simulink library "WECSim_Lib_PTOs"  (R2020b)
settings: Solver=VariableStepAuto  StartTime=0.0  StopTime=10.0  RelTol=1e-3
undefined symbols (not defined in the file or in its folder): constraint, pto, simu, X, Y, Z
libraries: nesl_utility x71, sm_lib x46, WECSim_Lib_Body_Elements x1
(part 3 of 3)

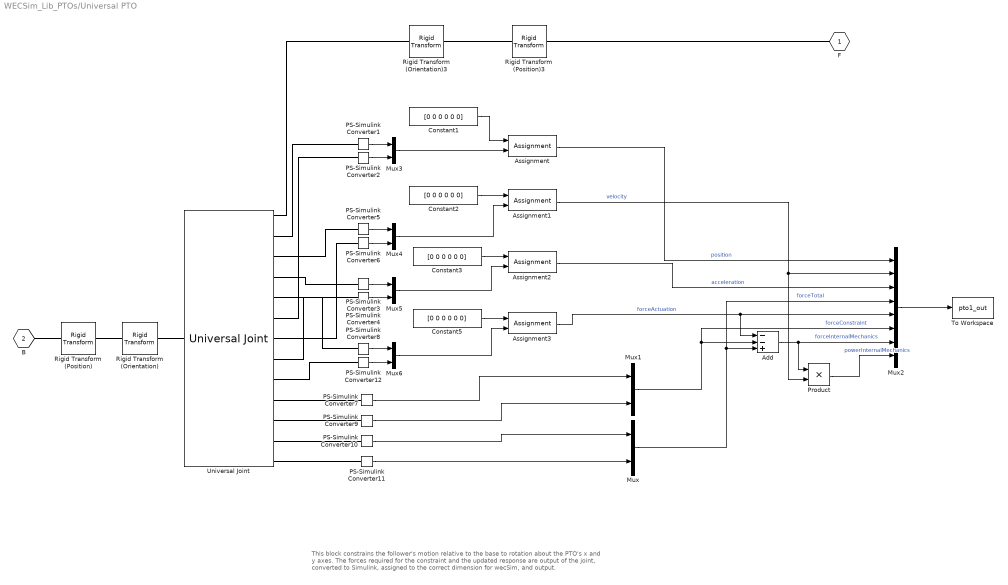
== system WECSim_Lib_PTOs/Universal PTO ==
  note: This block constrains the follower's motion relative to the base to rotation about the PTO's x and y axes. The forces required for the constraint and the updated response are output of the joint, converted to Simulink, assigned to the correct dimension for wecSim, and output.
  Add : Sum  Inputs=--+
  Assignment : Assignment  IndexOptions=Index vector (dialog)  Indices=[4 5]  OutputSizes=1
  Assignment1 : Assignment  IndexOptions=Index vector (dialog)  Indices=[4 5]  OutputSizes=1
  Assignment2 : Assignment  IndexOptions=Index vector (dialog)  Indices=[4,5]  OutputSizes=1
  Assignment3 : Assignment  IndexOptions=Index vector (dialog)  Indices=[4,5]  OutputSizes=1
  Constant{1..3,5} (4 alike) : Constant  Value=[0 0 0 0 0 0]
  Mux{,1,3..6} (6 alike) : Mux  Inputs=2
  Mux2 : Mux  Inputs=8
  PS-Simulink Converter{1..12} (12 alike) : nesl_utility/PS-Simulink Converter  PhysicalDomain=network_engine_domain  SubClassName=ps_output  LeftPortType=input  RightPortType=output  PseudoPeriodic=off  Frequencies=[]  VectorFormat=1-D array  Unit=inherit  AffineConversion=off
  Product : Product
  Rigid Transform (Orientation) : sm_lib/Frames and Transforms/Rigid Transform  RotationMethod=RotationMatrix  FollAlignAxisA=+X  BaseAlignAxisA=+Y  FollAlignAxisB=+Y  BaseAlignAxisB=+Z  RotationStandardAxis=+Z  RotationAngle=0.0  RotationAngleUnits=deg  RotationArbitraryAxis=[0 0 1]  RotationSequenceAxes=FollowerAxes  RotationSequence=XYX  RotationSequenceAngles=[0 0 0]  RotationSequenceAnglesUnits=deg  RotationMatrix=pto.orientation.rotationMatrix  Quaternion=[1 0 0 0]  TranslationMethod=None  TranslationCartesianOffset=constraint.initial.displacement+constraint.location  TranslationCartesianOffsetUnits=m  TranslationStandardAxis=+Z  TranslationStandardOffset=0  TranslationStandardOffsetUnits=m  TranslationROffset=0  TranslationROffsetUnits=m  TranslationThetaOffset=0  TranslationThetaOffsetUnits=deg  TranslationZOffset=0  TranslationZOffsetUnits=m
  Rigid Transform (Orientation)3 : sm_lib/Frames and Transforms/Rigid Transform  RotationMethod=RotationMatrix  FollAlignAxisA=+X  BaseAlignAxisA=+Y  FollAlignAxisB=+Y  BaseAlignAxisB=+Z  RotationStandardAxis=+Z  RotationAngle=0.0  RotationAngleUnits=deg  RotationArbitraryAxis=[0 0 1]  RotationSequenceAxes=FollowerAxes  RotationSequence=XYX  RotationSequenceAngles=[0 0 0]  RotationSequenceAnglesUnits=deg  RotationMatrix=pto.orientation.rotationMatrix  Quaternion=[1 0 0 0]  TranslationMethod=None  TranslationCartesianOffset=constraint.initial.displacement+constraint.location  TranslationCartesianOffsetUnits=m  TranslationStandardAxis=+Z  TranslationStandardOffset=0  TranslationStandardOffsetUnits=m  TranslationROffset=0  TranslationROffsetUnits=m  TranslationThetaOffset=0  TranslationThetaOffsetUnits=deg  TranslationZOffset=0  TranslationZOffsetUnits=m
  Rigid Transform (Position) : sm_lib/Frames and Transforms/Rigid Transform  RotationMethod=None  FollAlignAxisA=+X  BaseAlignAxisA=+Y  FollAlignAxisB=+Y  BaseAlignAxisB=+Z  RotationStandardAxis=+Z  RotationAngle=0.0  RotationAngleUnits=deg  RotationArbitraryAxis=[0 0 1]  RotationSequenceAxes=FollowerAxes  RotationSequence=XYX  RotationSequenceAngles=[0 0 0]  RotationSequenceAnglesUnits=deg  RotationMatrix=[1 0 0; 0 1 0; 0 0 1]  Quaternion=[1 0 0 0]  TranslationMethod=Cartesian  TranslationCartesianOffset=pto.initial.displacement+pto.location  TranslationCartesianOffsetUnits=m  TranslationStandardAxis=+Z  TranslationStandardOffset=0  TranslationStandardOffsetUnits=m  TranslationROffset=0  TranslationROffsetUnits=m  TranslationThetaOffset=0  TranslationThetaOffsetUnits=deg  TranslationZOffset=0  TranslationZOffsetUnits=m
  Rigid Transform (Position)3 : sm_lib/Frames and Transforms/Rigid Transform  RotationMethod=None  FollAlignAxisA=+X  BaseAlignAxisA=+Y  FollAlignAxisB=+Y  BaseAlignAxisB=+Z  RotationStandardAxis=+Z  RotationAngle=0.0  RotationAngleUnits=deg  RotationArbitraryAxis=[0 0 1]  RotationSequenceAxes=FollowerAxes  RotationSequence=XYX  RotationSequenceAngles=[0 0 0]  RotationSequenceAnglesUnits=deg  RotationMatrix=[1 0 0; 0 1 0; 0 0 1]  Quaternion=[1 0 0 0]  TranslationMethod=Cartesian  TranslationCartesianOffset=pto.initial.displacement+pto.location  TranslationCartesianOffsetUnits=m  TranslationStandardAxis=+Z  TranslationStandardOffset=0  TranslationStandardOffsetUnits=m  TranslationROffset=0  TranslationROffsetUnits=m  TranslationThetaOffset=0  TranslationThetaOffsetUnits=deg  TranslationZOffset=0  TranslationZOffsetUnits=m
  To Workspace : ToWorkspace  VariableName=pto1_out  SaveFormat=Structure With Time  SampleTime=simu.dtOut
  Universal Joint : sm_lib/Joints/Universal Joint  JointMode=Normal  CompositeWrenchDir=BaseOnFollower  CompositeWrenchFrame=BaseFrame  SenseConstraintForce=on  SenseConstraintTorque=on  SenseTotalForce=on  SenseTotalTorque=on  RxPositionTargetSpecify=off  RxPositionTargetPriority=High  RxPositionTargetValue=pto.extension.PositionTargetValue(1)  RxPositionTargetValueUnits=deg  RxVelocityTargetSpecify=off  RxVelocityTargetPriority=High  RxVelocityTargetValue=0  RxVelocityTargetValueUnits=deg/s  RxEquilibriumPosition=0  RxEquilibriumPositionUnits=deg  RxSpringStiffness=pto.stiffness  RxSpringStiffnessUnits=N*m/deg  RxDampingCoefficient=pto.damping  RxDampingCoefficientUnits=N*m/(deg/s)  RxLowerLimitSpecify=off  RxLowerLimitBound=pto.hardstops.lowerLimitBound(1)  RxLowerLimitBoundUnits=deg  RxLowerLimitStiffness=pto.hardstops.lowerLimitStiffness(1)  RxLowerLimitStiffnessUnits=N*m/deg  RxLowerLimitDamping=pto.hardstops.lowerLimitDamping(1)  RxLowerLimitDampingUnits=N*m/(deg/s)  RxLowerLimitTransitionRegionWidth=pto.hardstops.lowerLimitTransitionRegion(1)  RxLowerLimitTransitionRegionWidthUnits=deg  RxUpperLimitSpecify=off  RxUpperLimitBound=pto.hardstops.upperLimitBound(1)  RxUpperLimitBoundUnits=deg  RxUpperLimitStiffness=pto.hardstops.upperLimitStiffness(1)  RxUpperLimitStiffnessUnits=N*m/deg  RxUpperLimitDamping=pto.hardstops.upperLimitDamping(1)  RxUpperLimitDampingUnits=N*m/(deg/s)  RxUpperLimitTransitionRegionWidth=pto.hardstops.upperLimitTransitionRegionWidth(1)  RxUpperLimitTransitionRegionWidthUnits=deg  RxTorqueActuationMode=NoTorque  RxMotionActuationMode=ComputedMotion  RxSensePosition=on  RxSenseVelocity=on  RxSenseAcceleration=on  RxSenseTorqueForce=on  RxSenseLowerLimitTorqueForce=off  RxSenseUpperLimitTorqueForce=off  RyPositionTargetSpecify=off  RyPositionTargetPriority=High  RyPositionTargetValue=pto.extension.PositionTargetValue(2)  RyPositionTargetValueUnits=deg  RyVelocityTargetSpecify=off  RyVelocityTargetPriority=High  RyVelocityTargetValue=0  RyVelocityTargetValueUnits=deg/s  RyEquilibriumPosition=0  RyEquilibriumPositionUnits=deg  RySpringStiffness=pto.stiffness  RySpringStiffnessUnits=N*m/deg  RyDampingCoefficient=pto.damping  RyDampingCoefficientUnits=N*m/(deg/s)  RyLowerLimitSpecify=off  RyLowerLimitBound=pto.hardstops.lowerLimitBound(2)  RyLowerLimitBoundUnits=deg  RyLowerLimitStiffness=pto.hardstops.lowerLimitStiffness(2)  RyLowerLimitStiffnessUnits=N*m/deg  RyLowerLimitDamping=pto.hardstops.lowerLimitDamping(2)  RyLowerLimitDampingUnits=N*m/(deg/s)  RyLowerLimitTransitionRegionWidth=pto.hardstops.lowerLimitTransitionRegion(2)  RyLowerLimitTransitionRegionWidthUnits=deg  RyUpperLimitSpecify=off  RyUpperLimitBound=pto.hardstops.upperLimitBound(2)  RyUpperLimitBoundUnits=deg  RyUpperLimitStiffness=pto.hardstops.upperLimitStiffness(2)  RyUpperLimitStiffnessUnits=N*m/deg  RyUpperLimitDamping=pto.hardstops.upperLimitDamping(2)  RyUpperLimitDampingUnits=N*m/(deg/s)  RyUpperLimitTransitionRegionWidth=pto.hardstops.upperLimitTransitionRegionWidth(2)  RyUpperLimitTransitionRegionWidthUnits=deg  RyTorqueActuationMode=NoTorque  RyMotionActuationMode=ComputedMotion  RySensePosition=on  RySenseVelocity=on  RySenseAcceleration=on  RySenseTorqueForce=on  RySenseLowerLimitTorqueForce=off  RySenseUpperLimitTorqueForce=off
  F : PMIOPort  Side=Right
  B : PMIOPort  Port=2  Side=Left
  wires:
  Product/1 -> Mux2/8  "powerInternalMechanics"
  Add/1 -> Mux2/7, Product/1  "forceInternalMechanics"
  Mux/1 -> Mux2/4, Add/3  "forceTotal"
  Assignment2/1 -> Mux2/3  "acceleration"
  PS-Simulink Converter11/1 -> Mux/2
  Constant3/1 -> Assignment2/1
  Assignment1/1 -> Mux2/2, Product/2  "velocity"
  Constant2/1 -> Assignment1/1
  Mux5/1 -> Assignment2/2
  Assignment/1 -> Mux2/1  "position"
  PS-Simulink Converter7/1 -> Mux1/1
  PS-Simulink Converter10/1 -> Mux/1
  Mux4/1 -> Assignment1/2
  PS-Simulink Converter9/1 -> Mux1/2
  Mux3/1 -> Assignment/2
  Constant1/1 -> Assignment/1
  Mux2/1 -> To Workspace/1
  Mux1/1 -> Add/2, Mux2/6  "forceConstraint"
  PS-Simulink Converter1/1 -> Mux3/1
  PS-Simulink Converter2/1 -> Mux3/2
  PS-Simulink Converter3/1 -> Mux5/1
  PS-Simulink Converter4/1 -> Mux5/2
  PS-Simulink Converter6/1 -> Mux4/2
  PS-Simulink Converter5/1 -> Mux4/1
  PS-Simulink Converter8/1 -> Mux6/1
  Constant5/1 -> Assignment3/1
  PS-Simulink Converter12/1 -> Mux6/2
  Mux6/1 -> Assignment3/2
  Assignment3/1 -> Add/1, Mux2/5  "forceActuation"
  connections:
  Universal Joint/LConn1 -- Rigid Transform (Orientation)/RConn1
  Rigid Transform (Orientation)3/LConn1 -- Rigid Transform (Position)3/RConn1
  Rigid Transform (Position)/LConn1 -- B/RConn1
  Universal Joint/RConn1 -- Rigid Transform (Orientation)3/RConn1
  Rigid Transform (Orientation)/LConn1 -- Rigid Transform (Position)/RConn1
  Rigid Transform (Position)3/LConn1 -- F/RConn1
  Universal Joint/RConn2 -- PS-Simulink Converter1/LConn1
  Universal Joint/RConn13 -- PS-Simulink Converter11/LConn1
  Universal Joint/RConn12 -- PS-Simulink Converter10/LConn1
  Universal Joint/RConn11 -- PS-Simulink Converter9/LConn1
  Universal Joint/RConn10 -- PS-Simulink Converter7/LConn1
  Universal Joint/RConn8 -- PS-Simulink Converter4/LConn1
  Universal Joint/RConn6 -- PS-Simulink Converter2/LConn1
  Universal Joint/RConn4 -- PS-Simulink Converter3/LConn1
  Universal Joint/RConn7 -- PS-Simulink Converter6/LConn1
  Universal Joint/RConn3 -- PS-Simulink Converter5/LConn1
  Universal Joint/RConn9 -- PS-Simulink Converter12/LConn1
  Universal Joint/RConn5 -- PS-Simulink Converter8/LConn1
